simulink model "upr_1_3"  (R2019a)
settings: Solver=VariableStepAuto  StartTime=0.0  StopTime=10.0  RelTol=1e-3
values from neighbouring files (symbols this model uses):
  Kp = 1    [1upr.m]    (also in upr_1.m)
  Td = 3    [1upr.m]    (also in PIDtun_CC.m = L*(0.37-0.37*tau)/(1-0.81*tau); PIDtun_ZN1.m = L/2; PIDtun_ZN2.m = 0.125*Tu; upr_1.m = 0.04)
  Ti = 0.5    [1upr.m]    (also in PIDtun_CC.m = L*(2.5-2*tau)/(1-0.39*tau); PIDtun_ZN1.m = 2*L; PIDtun_ZN2.m = 0.5*Tu; upr_1.m = 0.2)
undefined symbols (not defined in the file or in its folder): B, C, N
settings Model: Creator=user1  LastModifiedBy=user1

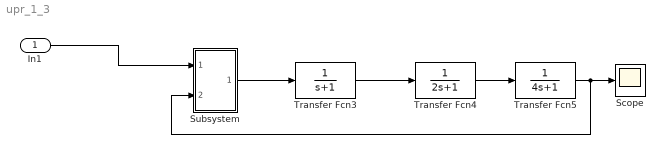
== system upr_1_3 ==
  In1 : Inport
  Scope : Scope
  Subsystem : Subsystem
  Transfer Fcn3 : TransferFcn  Denominator=[1 1]
  Transfer Fcn4 : TransferFcn  Denominator=[2 1]
  Transfer Fcn5 : TransferFcn  Denominator=[4 1]
  wires:
  In1/1 -> Subsystem/1(In1)
  Transfer Fcn4/1 -> Transfer Fcn5/1
  Transfer Fcn3/1 -> Transfer Fcn4/1
  Subsystem/1(Out1) -> Transfer Fcn3/1
  Transfer Fcn5/1 -> Subsystem/2(In2), Scope/1

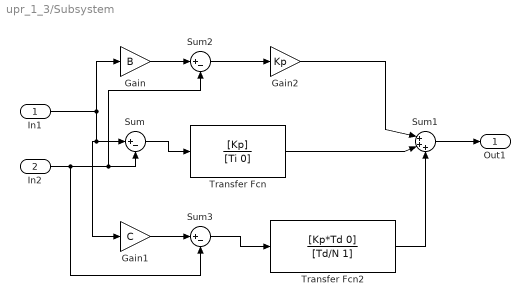
== system upr_1_3/Subsystem ==
  In1 : Inport
  In2 : Inport  Port=2
  Gain : Gain  Gain=B
  Gain1 : Gain  Gain=C
  Gain2 : Gain  Gain=Kp
  Sum : Sum  Inputs=|+-
  Sum1 : Sum  Inputs=|+++
  Sum2 : Sum  Inputs=|+-
  Sum3 : Sum  Inputs=|+-
  Transfer Fcn : TransferFcn  Numerator=[Kp]  Denominator=[Ti 0]
  Transfer Fcn2 : TransferFcn  Numerator=[Kp*Td 0]  Denominator=[Td/N 1]
  Out1 : Outport
  wires:
  Transfer Fcn2/1 -> Sum1/3
  Sum1/1 -> Out1/1
  Sum3/1 -> Transfer Fcn2/1
  In2/1 -> Sum3/2, Sum2/2, Sum/2
  Gain/1 -> Sum2/1
  Gain1/1 -> Sum3/1
  Sum/1 -> Transfer Fcn/1
  Transfer Fcn/1 -> Sum1/2
  Gain2/1 -> Sum1/1
  In1/1 -> Gain1/1, Sum/1, Gain/1
  Sum2/1 -> Gain2/1
